simulink model "lab8"  (R2013b)
settings: Solver=ode3  StartTime=0.0  StopTime=30  FixedStep=0.01  RelTol=1e-3
settings Model: Creator=Niirn  LastModifiedBy=Niirn

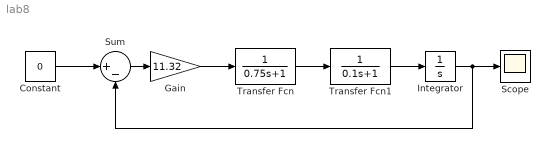
== system lab8 ==
  Constant : Constant  Value=0
  Gain : Gain  Gain=11.32
  Integrator : Integrator  InitialCondition=1
  Scope : Scope
  Sum : Sum  Inputs=|+-
  Transfer Fcn : TransferFcn  Denominator=[0.75 1]
  Transfer Fcn1 : TransferFcn  Denominator=[0.1 1]
  wires:
  Transfer Fcn1/1 -> Integrator/1
  Transfer Fcn/1 -> Transfer Fcn1/1
  Gain/1 -> Transfer Fcn/1
  Sum/1 -> Gain/1
  Constant/1 -> Sum/1
  Integrator/1 -> Scope/1, Sum/2
